simulink model "QuadcopterSimModel_LindiCopter"  (R2018b)
settings: Solver=ode23  StartTime=0.0  StopTime=1000  FixedStep=sample_time  RelTol=1e-4  EnableMultiTasking=on
undefined symbols (not defined in the file): alt_ground, atmosphere, envir, g, G10, G20, joystick, lindi, pos_ref, waypoints, wind
libraries: filters_lib x8, indi_lib x3, unit_conversions_lib x3, simulink x2, flightgear_visualization_lib x2, axes_transformation_lib x2, cntrlPosNdi_lib x2, atmosphere_lib x1, ca_lib x1, ndi_lib x1, traj_lib x1, cntrlAttiRedIndi_lib x1
settings Model: EnablePacing=on  Creator=Yannic  LastModifiedBy=yannic
settings SolverCC: ZeroCrossControl=DisableAll
settings DataIOCC: LimitDataPoints=on  ReturnWorkspaceOutputs=on
settings OptimizationCC: EfficientMapNaN2IntZero=off  LifeSpan=inf
settings DebuggingCC: ReadBeforeWriteMsg=DisableAll  WriteAfterWriteMsg=DisableAll  WriteAfterReadMsg=DisableAll  MultiTaskDSMMsg=none  AllowSymbolicDim=off  LibraryContextMissingDiagnostic=none  SFUnexpectedBacktrackingDiag=warning  SFNoUnconditionalDefaultTransitionDiag=warning  SFExecutionAtInitializationDiag=none
settings HardwareCC: TargetBitPerLong=64  TargetBitPerPointer=64  TargetBitPerSizeT=64  TargetBitPerPtrDiffT=64  TargetLongLongMode=on  TargetIntDivRoundTo=Zero  TargetEndianess=LittleEndian  TargetWordSize=64  TargetHWDeviceType=MATLAB Host  ProdEqTarget=off
settings ModelReferenceCC: UpdateModelReferenceTargets=IfOutOfDate  PropagateSignalLabelsOutOfModel=off
settings SFSimCC: SFSimEcho=off  SimUseLocalCustomCode=off
settings CodeAppCC: MaxIdLength=128
settings GRTTargetCC: TargetLangStandard=C89/C90 (ANSI)  CombineOutputUpdateFcns=off  GRTInterface=on
settings ConfigComp: CovMetricSettings=dw  CovHtmlReporting=on  CovSaveCumulativeToWorkspaceVar=on  CovSaveSingleToWorkspaceVar=on  CovExternalEMLEnable=off

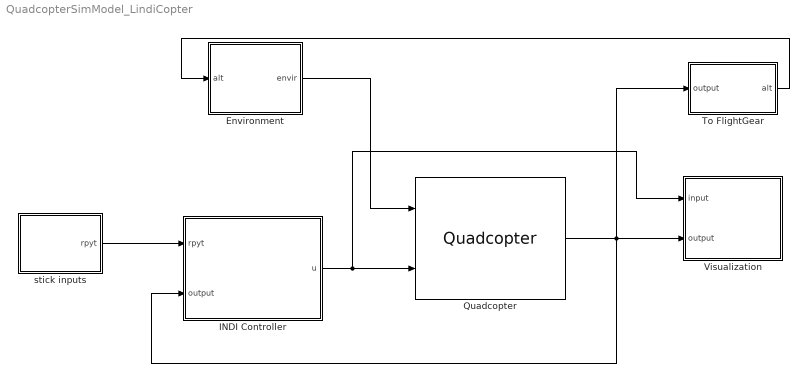
== system QuadcopterSimModel_LindiCopter ==
  Environment : Subsystem
  INDI Controller : Subsystem
  Quadcopter : quadcopter_lib/Quadcopter  copter_=copter  IC_=IC  grnd_=grnd
      settings: SourceProductName=LADAC
  To FlightGear : Subsystem
  Visualization : Subsystem
  stick inputs : Subsystem
  wires:
  Environment/1(envir) -> Quadcopter/1
  Quadcopter/1 -> To FlightGear/1(output), Visualization/2(output), INDI Controller/2(output)
  To FlightGear/1(alt) -> Environment/1(alt)
  INDI Controller/1(u) -> Quadcopter/2, Visualization/1(input)
  stick inputs/1(rpyt) -> INDI Controller/1(rpyt)

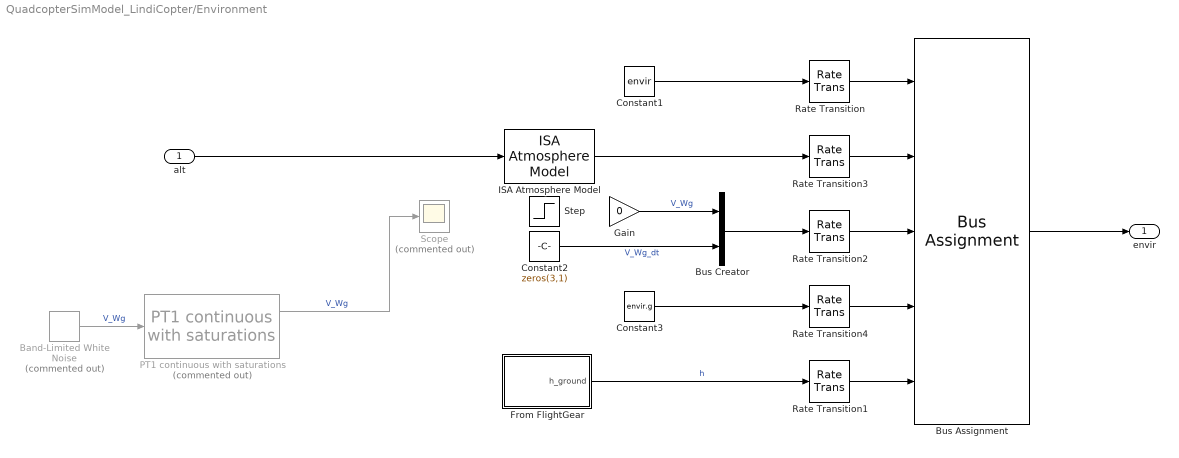
== system QuadcopterSimModel_LindiCopter/Environment ==
  alt : Inport
  Band-Limited White Noise : simulink/Sources/Band-Limited White Noise  Commented=on  Cov=10  Ts=0.0025  seed=[23341,12345,23456]
  Bus Assignment : BusAssignment  AssignedSignals=atmosphere,wind,g,alt_ground
  Bus Creator : BusCreator  Inputs=2
  Constant1 : Constant  Value=envir  OutDataTypeStr=Bus: envirBus
  Constant2 : Constant  Value=zeros(3,1)
  Constant3 : Constant  Value=envir.g
  From FlightGear : Subsystem
  Gain : Gain  Gain=0
  ISA Atmosphere Model : atmosphere_lib/ISA Atmosphere Model
      settings: SourceProductName=LADAC
  PT1 continuous with saturations : filters_lib/PT1 continuous with saturations  Commented=on  T=0.5  x_max=inf  x_min=-inf  x_dt_max=inf  x_dt_min=-inf  x_init=0
      settings: SourceProductName=LADAC
  Rate Transition{,1..4} (5 alike) : RateTransition
  Scope : Scope  Commented=on
  Step : Step  Time=5  After=[0;10;0]  SampleTime=0
  envir : Outport
  wires:
  From FlightGear/1(h_ground) -> Rate Transition1/1  "h"
  Rate Transition2/1 -> Bus Assignment/3
  Rate Transition3/1 -> Bus Assignment/2
  Bus Assignment/1 -> envir/1
  Rate Transition/1 -> Bus Assignment/1
  ISA Atmosphere Model/1 -> Rate Transition3/1
  PT1 continuous with saturations/1 -> Scope/1  "V_Wg"
  Rate Transition1/1 -> Bus Assignment/5
  Constant1/1 -> Rate Transition/1
  alt/1 -> ISA Atmosphere Model/1
  Bus Creator/1 -> Rate Transition2/1
  Constant2/1 -> Bus Creator/2  "V_Wg_dt"
  Rate Transition4/1 -> Bus Assignment/4
  Constant3/1 -> Rate Transition4/1
  Gain/1 -> Bus Creator/1  "V_Wg"
  Band-Limited White Noise/1 -> PT1 continuous with saturations/1  "V_Wg"

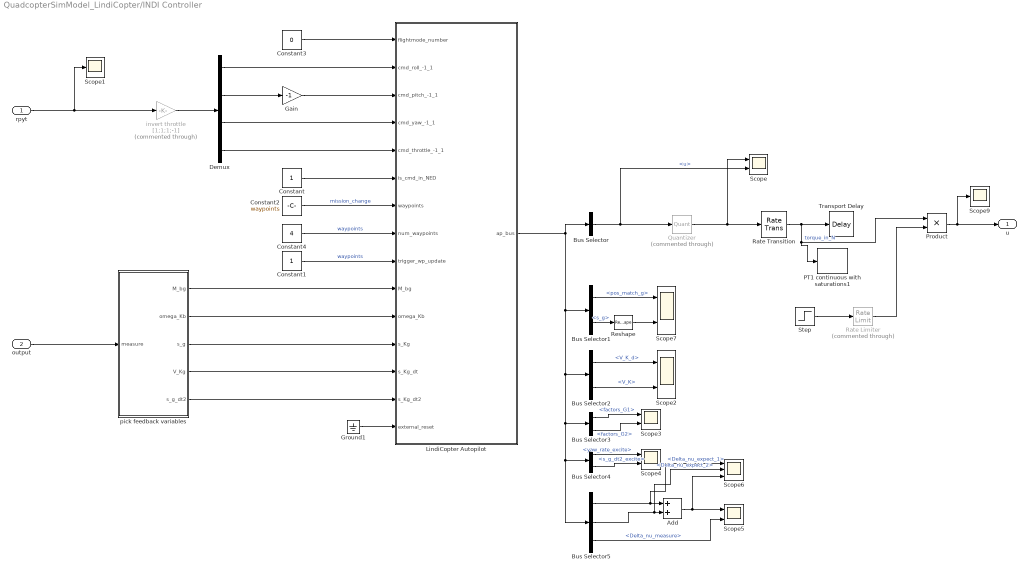
== system QuadcopterSimModel_LindiCopter/INDI Controller ==
  rpyt : Inport  OutDataTypeStr=double
  output : Inport  Port=2
  Add : Sum
  Bus Selector : BusSelector  OutputSignals=inner_loop_indi.u
  Bus Selector1 : BusSelector  OutputSignals=guidance.matching.pos_match_g,pos_cntrl.measure.s_g
  Bus Selector2 : BusSelector  OutputSignals=guidance.velocity.V_K_d,guidance.velocity.V_K
  Bus Selector3 : BusSelector  OutputSignals=autotune.factors_G1,autotune.factors_G2
  Bus Selector4 : BusSelector  OutputSignals=autotune.excite.yaw_rate_excite,autotune.excite.s_g_dt2_excite
  Bus Selector5 : BusSelector  OutputSignals=autotune.indi_inv_check.Delta_nu_expect_1,autotune.indi_inv_check.Delta_nu_expect_2,autotune.indi_inv_check.Delta_nu_measure
  Constant : Constant
  Constant1 : Constant
  Constant2 : Constant  Value=waypoints
  Constant3 : Constant  Value=0
  Constant4 : Constant  Value=4
  Demux : Demux
  Gain : Gain  Gain=-1
  Ground1 : Ground
  LindiCopter Autopilot : Subsystem  AncestorBlock=lindiCopter_lib/LindiCopter Autopilot  mask{ap=lindi}
      mask prompts: ap "LinidCopter parameters struct, see lindiCopter_params_default"
      mask init:
      | lindiCopterStateLogicBus();
      mask Help: web('hhttps://github.com/iff-gsc/LADAC/tree/main/control/autopilots/LindiCopter/README.md','-browser')
      mask DialogControl DescGroupVar Prompt: LindiCopter Autopilot
      mask DialogControl Control4 Prompt: The documentation of this block can be found here:
      mask DialogControl Control5 Prompt: README
      mask DialogControl Control5 Callback: web('https://github.com/iff-gsc/LADAC/blob/main/control/autopilots/LindiCopter/README.md','-browser')
  PT1 continuous with saturations1 : filters_lib/PT1 continuous with saturations  T=0.03  x_max=inf  x_min=-inf  x_dt_max=inf  x_dt_min=-inf  x_init=0
      settings: SourceProductName=LADAC
  Product : Product
  Quantizer : Quantizer  Commented=through  QuantizationInterval=0.001
  Rate Limiter : RateLimiter  Commented=through  RisingSlewLimit=0.3  FallingSlewLimit=-0.3  SampleTimeMode=inherited
  Rate Transition : RateTransition
  Reshape : Reshape
  Scope{,2..5,7} (6 alike) : Scope  NumInputPorts=2
  Scope1 : Scope
  Scope6 : Scope  NumInputPorts=3
  Scope9 : Scope
  Step : Step  Time=0  Before=[1;1;1;1]  After=[1;0;1;1]  SampleTime=0
  Transport Delay : TransportDelay  DelayTime=0.0025*2
  invert throttle : Gain  Commented=through  Gain=[1;1;1;-1]
  pick feedback variables : Subsystem
  u : Outport  OutDataTypeStr=double  PortDimensions=4
  wires:
  output/1 -> pick feedback variables/1(measure)
  rpyt/1 -> invert throttle/1, Scope1/1
  Bus Selector/1 -> Quantizer/1, Scope/2  "<u>"
  invert throttle/1 -> Demux/1
  LindiCopter Autopilot/1(ap_bus) -> Bus Selector/1, Bus Selector5/1, Bus Selector4/1, Bus Selector3/1, Bus Selector2/1, Bus Selector1/1
  Demux/4 -> LindiCopter Autopilot/5(cmd_throttle_-1_1)
  Demux/3 -> LindiCopter Autopilot/4(cmd_yaw_-1_1)
  Constant/1 -> LindiCopter Autopilot/6(is_cmd_in_NED)
  Ground1/1 -> LindiCopter Autopilot/15(external_reset)
  Demux/2 -> Gain/1
  Demux/1 -> LindiCopter Autopilot/2(cmd_roll_-1_1)
  Gain/1 -> LindiCopter Autopilot/3(cmd_pitch_-1_1)
  pick feedback variables/1(M_bg) -> LindiCopter Autopilot/10(M_bg)
  pick feedback variables/2(omega_Kb) -> LindiCopter Autopilot/11(omega_Kb)
  pick feedback variables/3(s_g) -> LindiCopter Autopilot/12(s_Kg)
  pick feedback variables/4(V_Kg) -> LindiCopter Autopilot/13(s_Kg_dt)
  Constant1/1 -> LindiCopter Autopilot/9(trigger_wp_update)  "waypoints"
  Constant2/1 -> LindiCopter Autopilot/7(waypoints)  "mission_change"
  Bus Selector1/2 -> Reshape/1  "<s_g>"
  Bus Selector1/1 -> Scope7/1  "<pos_match_g>"
  Bus Selector2/2 -> Scope2/2  "<V_K>"
  Bus Selector2/1 -> Scope2/1  "<V_K_d>"
  Constant3/1 -> LindiCopter Autopilot/1(flightmode_number)
  Quantizer/1 -> Rate Transition/1, Scope/1
  pick feedback variables/5(s_g_dt2) -> LindiCopter Autopilot/14(s_Kg_dt2)
  Reshape/1 -> Scope7/2
  Bus Selector3/1 -> Scope3/1  "<factors_G1>"
  Bus Selector3/2 -> Scope3/2  "<factors_G2>"
  Bus Selector4/1 -> Scope4/1  "<yaw_rate_excite>"
  Bus Selector4/2 -> Scope4/2  "<s_g_dt2_excite>"
  Bus Selector5/1 -> Scope6/1, Add/1  "<Delta_nu_expect_1>"
  Bus Selector5/2 -> Scope6/2, Add/2  "<Delta_nu_expect_2>"
  Add/1 -> Scope6/3, Scope5/1
  Bus Selector5/3 -> Scope5/2  "<Delta_nu_measure>"
  Step/1 -> Rate Limiter/1
  Constant4/1 -> LindiCopter Autopilot/8(num_waypoints)  "waypoints"
  Product/1 -> Scope9/1, u/1
  Rate Transition/1 -> Product/1, PT1 continuous with saturations1/1, Transport Delay/1  "torque_in_N"
  Rate Limiter/1 -> Product/2

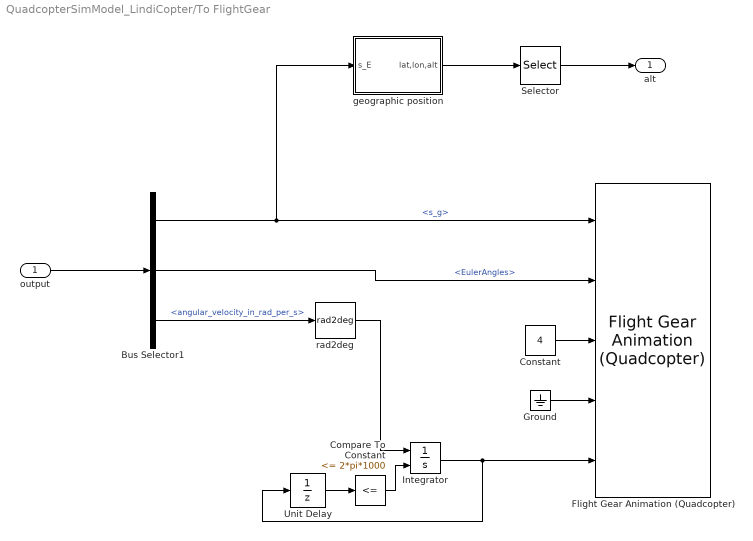
== system QuadcopterSimModel_LindiCopter/To FlightGear ==
  output : Inport
  Bus Selector1 : BusSelector  OutputSignals=rigidBodyBus.s_g,rigidBodyBus.EulerAngles,motorBus.angular_velocity_in_rad_per_s
  Compare To Constant : simulink/Logic and Bit Operations/Compare To Constant  relop=<=  const=2*pi*1000  OutDataTypeStr=boolean
  Constant : Constant  Value=4
  Flight Gear Animation (Quadcopter) : flightgear_visualization_lib/Flight Gear Animation (Quadcopter)  inital_lat=pos_ref.lat  inital_long=pos_ref.lon  inital_height=pos_ref.alt  remoteURL=fg.remoteURL  remotePort=fg.remotePort
      settings: SourceProductName=LADAC
  Ground : Ground
  Integrator : Integrator  ExternalReset=rising
  Selector : Selector  InputPortWidth=3  IndexOptions=Index vector (dialog)  Indices=3  OutputSizes=1
  Unit Delay : UnitDelay  SampleTime=-1
  geographic position : Subsystem
  rad2deg : unit_conversions_lib/rad2deg
      settings: SourceProductName=LADAC
  alt : Outport
  wires:
  Bus Selector1/1 -> geographic position/1(s_E), Flight Gear Animation (Quadcopter)/1  "<s_g>"
  output/1 -> Bus Selector1/1
  geographic position/1(lat,lon,alt) -> Selector/1
  Bus Selector1/2 -> Flight Gear Animation (Quadcopter)/2  "<EulerAngles>"
  Bus Selector1/3 -> rad2deg/1  "<angular_velocity_in_rad_per_s>"
  Selector/1 -> alt/1
  Constant/1 -> Flight Gear Animation (Quadcopter)/3
  Ground/1 -> Flight Gear Animation (Quadcopter)/4
  Integrator/1 -> Unit Delay/1, Flight Gear Animation (Quadcopter)/5
  Unit Delay/1 -> Compare To Constant/1
  Compare To Constant/1 -> Integrator/2
  rad2deg/1 -> Integrator/1

== system QuadcopterSimModel_LindiCopter/Visualization ==
  input : Inport
  output : Inport  Port=2
  Aerodynamics : Subsystem
  Bus Selector : BusSelector  OutputSignals=rigidBodyBus,aeroBus,propulsionBus,motorBus
  Motor : Subsystem
  Propulsion : Subsystem
  Scope : Scope
  rigid_body : Subsystem
  wires:
  output/1 -> Bus Selector/1
  Bus Selector/1 -> rigid_body/1(rigidBodyBus)  "<rigidBodyBus>"
  Bus Selector/2 -> Aerodynamics/1(aeroBus)  "<aeroBus>"
  Bus Selector/3 -> Propulsion/1(propulsionBus)  "<propulsionBus>"
  Bus Selector/4 -> Motor/1(motorBus)  "<motorBus>"
  input/1 -> Scope/1

== system QuadcopterSimModel_LindiCopter/stick inputs ==
  Calibrated Joystick : joystick_lib/Calibrated Joystick  jystck=joystick  joyid=1
      settings: SourceProductName=LADAC
  Constant : Constant  Value=zeros(8,1)
  Constant1 : Constant  Value=joystick.enable
  Scope : Scope
  Selector2 : Selector  InputPortWidth=8  IndexOptions=Index vector (dialog)  Indices=[1,2,3,4]  OutputSizes=1
  Switch1 : Switch  Criteria=u2 > Threshold
  rpyt : Outport
  wires:
  Constant/1 -> Switch1/3
  Switch1/1 -> Selector2/1, Scope/1
  Constant1/1 -> Calibrated Joystick/Enable, Switch1/2
  Calibrated Joystick/1 -> Switch1/1
  Selector2/1 -> rpyt/1

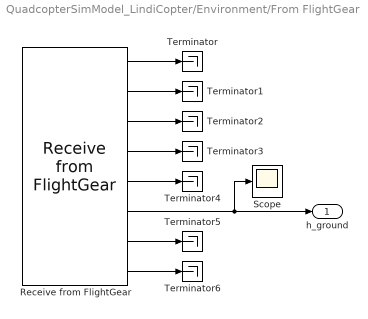
== system QuadcopterSimModel_LindiCopter/Environment/From FlightGear ==
  Receive from FlightGear : flightgear_visualization_lib/Receive from FlightGear  ip_address='127.0.0.1'  ip_port=5503  sample_time=1/30  blocking_time=0  is_aerocntrl=off  is_engine=off  is_fuel=off  is_land=off  is_avionics=off  is_envir=on
      settings: SourceProductName=LADAC
  Scope : Scope
  Terminator{,1..6} (7 alike) : Terminator
  h_ground : Outport
  wires:
  Receive from FlightGear/4 -> Terminator3/1
  Receive from FlightGear/5 -> Terminator4/1
  Receive from FlightGear/2 -> Terminator1/1
  Receive from FlightGear/7 -> Terminator5/1
  Receive from FlightGear/1 -> Terminator/1
  Receive from FlightGear/3 -> Terminator2/1
  Receive from FlightGear/8 -> Terminator6/1
  Receive from FlightGear/6 -> Scope/1, h_ground/1

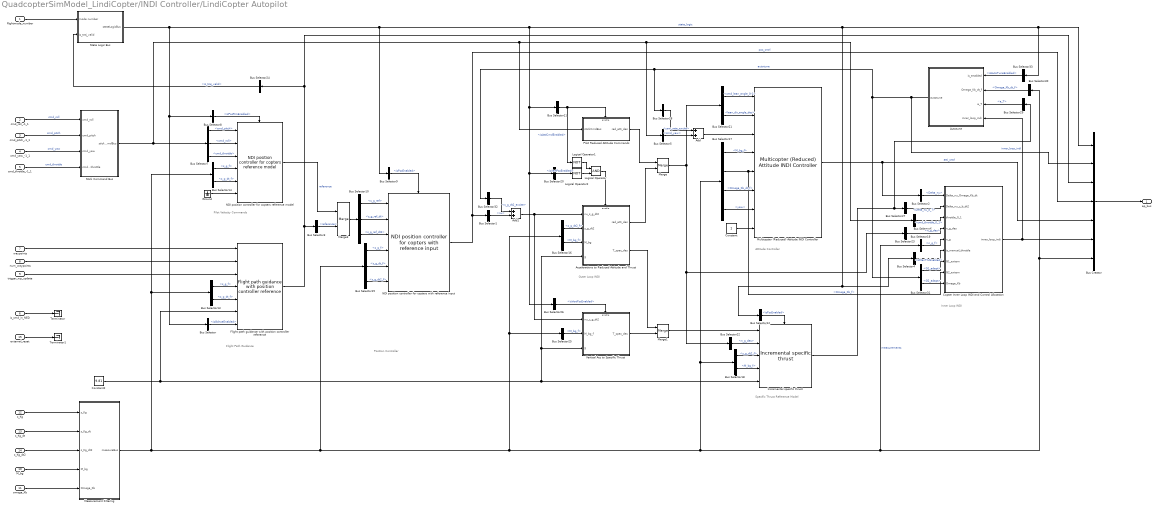
== system QuadcopterSimModel_LindiCopter/INDI Controller/LindiCopter Autopilot ==
  note: Inner Loop INDI
  note: Attitude Controller
  note: Specific Thrust
      | Reference Model
  note: Outer Loop INDI
  note: Pilot Velocity Commands
  note: Flight Path Guidance
  note: Position Controller
  flightmode_number : Inport  SampleTime=ap.ts
  cmd_roll_-1_1 : Inport  Port=2  SampleTime=ap.ts
  cmd_pitch_-1_1 : Inport  Port=3  SampleTime=ap.ts
  cmd_yaw_-1_1 : Inport  Port=4  SampleTime=ap.ts
  cmd_throttle_-1_1 : Inport  Port=5  SampleTime=ap.ts
  is_cmd_in_NED : Inport  Port=6  SampleTime=ap.ts
  waypoints : Inport  Port=7  SampleTime=ap.ts
  num_waypoints : Inport  Port=8  SampleTime=ap.ts
  trigger_wp_update : Inport  Port=9  SampleTime=ap.ts
  M_bg : Inport  Port=10  SampleTime=ap.ts
  omega_Kb : Inport  Port=11  SampleTime=ap.ts
  s_Kg : Inport  Port=12  SampleTime=ap.ts
  s_Kg_dt : Inport  Port=13  SampleTime=ap.ts
  s_Kg_dt2 : Inport  Port=14  SampleTime=ap.ts
  external_reset : Inport  Port=15  SampleTime=ap.ts
  Accelerations to Reduced Attitude and Thrust : Subsystem
  Add : Sum
  Add1 : Sum
  Autotune : Subsystem
  Bus Creator : BusCreator  Inputs=7
  Bus Selector : BusSelector  OutputSignals=isGdnceEnabled
  Bus Selector1 : BusSelector  OutputSignals=pseudo_control.nu
  Bus Selector10 : BusSelector  OutputSignals=s_g_ref,s_g_ref_dt,s_g_ref_dt2
  Bus Selector11 : BusSelector  OutputSignals=isAttiCmdEnabled
  Bus Selector12 : BusSelector  OutputSignals=isPscEnabled
  Bus Selector13 : BusSelector  OutputSignals=s_g_f,s_g_dt_f
  Bus Selector14 : BusSelector  OutputSignals=s_g_f,s_g_dt_f
  Bus Selector15 : BusSelector  OutputSignals=s_g_f,s_g_dt_f,s_g_dt2_f
  Bus Selector16 : BusSelector  OutputSignals=s_g_dt2_f,M_bg_f
  Bus Selector17 : BusSelector  OutputSignals=M_bg_f,Omega_Kb_f,Omega_Kb_dt_f,yaw
  Bus Selector18 : BusSelector  OutputSignals=s_g_dt2_f,M_bg_f
  Bus Selector19 : BusSelector  OutputSignals=n_g_f
  Bus Selector2 : BusSelector  OutputSignals=pseudo_control.Delta_ny
  Bus Selector20 : BusSelector  OutputSignals=isVertPscEnabled
  Bus Selector21 : BusSelector  OutputSignals=cmd_lean_angle_0-1,lean_dir_angle_des
  Bus Selector22 : BusSelector  OutputSignals=n_g_des
  Bus Selector23 : BusSelector  OutputSignals=n_g_des
  Bus Selector24 : BusSelector  OutputSignals=is_traj_valid
  Bus Selector25 : BusSelector  OutputSignals=M_bg_f
  Bus Selector26 : BusSelector  OutputSignals=isVertPscEnabled
  Bus Selector27 : BusSelector  OutputSignals=Delta_nu_a_T
  Bus Selector28 : BusSelector  OutputSignals=excite.yaw_rate_excite
  Bus Selector29 : BusSelector  OutputSignals=a_T
  Bus Selector3 : BusSelector  OutputSignals=reference
  Bus Selector30 : BusSelector  OutputSignals=Omega_Kb_dt_f
  Bus Selector31 : BusSelector  OutputSignals=G1_adapt,G2_adapt
  Bus Selector32 : BusSelector  OutputSignals=excite.s_g_dt2_excite
  Bus Selector33 : BusSelector  OutputSignals=isAutoTuneEnabled
  Bus Selector4 : BusSelector  OutputSignals=isManThrEnabled
  Bus Selector5 : BusSelector  OutputSignals=cmd_yaw
  Bus Selector6 : BusSelector  OutputSignals=cmd_throttle_0_1
  Bus Selector7 : BusSelector  OutputSignals=cmd_pitch,cmd_roll,cmd_throttle
  Bus Selector8 : BusSelector  OutputSignals=isPosRmEnabled
  Bus Selector9 : BusSelector  OutputSignals=isPscEnabled
  Constant : Constant
  Constant2 : Constant  Value=9.81
  Copter Inner Loop INDI and Control Allocation : Subsystem  AncestorBlock=indi_lib/Copter Inner Loop INDI and Control Allocation  mask{cep=ap.cep, ceb=ap.ceb, ca=ap.ca, mtc=ap.mtc, sflt=ap.sflt, ts=ap.ts, is_ce_extern=on}
      mask prompts: cep "Parameters for motor-propeller control effectiveness, see indiCeProp_params_default"; ceb "Parameters for body control effectiveness, see indiCeBody_params_default"; ca "Control allocation parameters, see controlAllocationWlsLoadParams"; mtc "Motor time constant, s"; sflt "Sensor filter parameters, see indiSensFiltLoadParams"; ts "Sample time, s"; is_ce_extern "Enable external control effectiveness"
      mask init:
      | caIndiCopterBlockInit(is_ce_extern);
      mask DialogControl DescGroupVar Prompt: Copter Inner Loop INDI and Control Allocation
  Flight path guidance with position controller reference : traj_lib/Flight path guidance with position controller reference  traj_params=ap.traj  T_inner_loop=2./ap.atc.rm.leanfreq + ap.mtc + 2./ap.sflt.omega
      settings: SourceProductName=LADAC
  Ground : Ground
  Incremental specific thrust : indi_lib/Incremental specific thrust  leanfreq=ap.atc.rm.leanfreq  leandamp=ap.atc.rm.leandamp  is_enable_checked=on  states_when_enabling=held
      settings: SourceProductName=LADAC
  Logical Operator : Logic  AllPortsSameDT=off  OutDataTypeStr=boolean
  Logical Operator1 : Logic  Operator=NOT  AllPortsSameDT=off  OutDataTypeStr=boolean
  Logical Operator2 : Logic  Operator=NOT  AllPortsSameDT=off  OutDataTypeStr=boolean
  Measurement Filtering : Subsystem
  Merge : Merge
  Merge1 : Merge
  Merge3 : Merge
  Multicopter (Reduced) Attitude INDI Controller : cntrlAttiRedIndi_lib/Multicopter (Reduced) Attitude INDI Controller  atc=ap.atc  T=ap.mtc + 2./ap.sflt.omega
      settings: SourceProductName=LADAC
  NDI position controller for copters reference model : cntrlPosNdi_lib/NDI position controller for copters reference model  psc=ap.psc  is_enable_checked=on  states_when_enabling=reset
      settings: SourceProductName=LADAC
  NDI position controller for copters with reference input : cntrlPosNdi_lib/NDI position controller for copters with reference input  psc=ap.psc  T_inner_loop=2./ap.atc.rm.leanfreq + ap.mtc + 2./ap.sflt.omega  is_enable_checked=on  states_when_enabling=held
      settings: SourceProductName=LADAC
  Pilot Reduced Attitude Commands : Subsystem
  State Logic Bus : Subsystem
  Stick Command Bus : Subsystem
  Terminator : Terminator
  Terminator1 : Terminator
  Vertical Acc to Specific Thrust : Subsystem
  ap_bus : Outport  SampleTime=ap.ts
  wires:
  num_waypoints/1 -> Flight path guidance with position controller reference/2
  Bus Selector5/1 -> Add/2  "<cmd_yaw>"
  Bus Selector33/1 -> Autotune/1(is_enabled)  "<isAutoTuneEnabled>"
  Bus Selector32/1 -> Add1/1  "<s_g_dt2_excite>"
  Bus Selector28/1 -> Add/1  "<yaw_rate_excite>"
  Autotune/1(autotune) -> Bus Selector32/1, Bus Selector28/1, Bus Selector31/1, Bus Creator/2  "autotune"
  Bus Selector29/1 -> Autotune/3(a_T)  "<a_T>"
  Bus Selector30/1 -> Autotune/2(Omega_Kb_dt_f)  "<Omega_Kb_dt_f>"
  Bus Selector31/1 -> Copter Inner Loop INDI and Control Allocation/7(G1_extern)  "<G1_adapt>"
  Bus Selector31/2 -> Copter Inner Loop INDI and Control Allocation/8(G2_extern)  "<G2_adapt>"
  Bus Selector27/1 -> Copter Inner Loop INDI and Control Allocation/2(Delta_nu_z_b_dt2)  "<Delta_nu_a_T>"
  Logical Operator/1 -> Accelerations to Reduced Attitude and Thrust/Enable
  Logical Operator2/1 -> Logical Operator/2
  Logical Operator1/1 -> Logical Operator/1
  Bus Selector26/1 -> Vertical Acc to Specific Thrust/Enable  "<isVertPscEnabled>"
  Bus Selector25/1 -> Vertical Acc to Specific Thrust/2(M_bg_f)  "<M_bg_f>"
  Vertical Acc to Specific Thrust/1(T_spec_des) -> Merge1/2
  Accelerations to Reduced Attitude and Thrust/2(T_spec_des) -> Merge1/1
  Accelerations to Reduced Attitude and Thrust/1(red_atti_des) -> Merge/2
  Bus Selector23/1 -> Copter Inner Loop INDI and Control Allocation/4(n_g_des)  "<n_g_des>"
  Pilot Reduced Attitude Commands/1(red_atti_des) -> Merge/1
  Merge/1 -> Bus Selector23/1, Bus Selector22/1, Bus Selector21/1
  Bus Selector21/2 -> Multicopter (Reduced) Attitude INDI Controller/2  "<lean_dir_angle_des>"
  Bus Selector21/1 -> Multicopter (Reduced) Attitude INDI Controller/1  "<cmd_lean_angle_0-1>"
  cmd_throttle_-1_1/1 -> Stick Command Bus/4(cmd_throttle)  "cmd_throttle"
  cmd_yaw_-1_1/1 -> Stick Command Bus/3(cmd_yaw)  "cmd_yaw"
  cmd_pitch_-1_1/1 -> Stick Command Bus/2(cmd_pitch)  "cmd_pitch"
  cmd_roll_-1_1/1 -> Stick Command Bus/1(cmd_roll)  "cmd_roll"
  Stick Command Bus/1(stickCmdBus) -> Bus Selector7/1, Bus Selector5/1, Bus Selector6/1, Pilot Reduced Attitude Commands/1(stickCmdBus)
  Bus Selector17/4 -> Multicopter (Reduced) Attitude INDI Controller/7  "<yaw>"
  Bus Selector19/1 -> Copter Inner Loop INDI and Control Allocation/5(n_g)  "<n_g_f>"
  Bus Selector22/1 -> Incremental specific thrust/2  "<n_g_des>"
  Bus Selector18/2 -> Incremental specific thrust/4  "<M_bg_f>"
  Bus Selector18/1 -> Incremental specific thrust/3  "<s_g_dt2_f>"
  Bus Selector17/3 -> Multicopter (Reduced) Attitude INDI Controller/6  "<Omega_Kb_dt_f>"
  Bus Selector17/2 -> Copter Inner Loop INDI and Control Allocation/9(Omega_Kb), Multicopter (Reduced) Attitude INDI Controller/5  "<Omega_Kb_f>"
  Bus Selector17/1 -> Multicopter (Reduced) Attitude INDI Controller/4  "<M_bg_f>"
  Bus Selector16/2 -> Accelerations to Reduced Attitude and Thrust/3(M_bg)  "<M_bg_f>"
  Bus Selector16/1 -> Accelerations to Reduced Attitude and Thrust/2(s_g_dt2)  "<s_g_dt2_f>"
  Bus Selector15/3 -> NDI position controller for copters with reference input/6  "<s_g_dt2_f>"
  Bus Selector15/2 -> NDI position controller for copters with reference input/5  "<s_g_dt_f>"
  Bus Selector15/1 -> NDI position controller for copters with reference input/4  "<s_g_f>"
  Bus Selector14/2 -> NDI position controller for copters reference model/5  "<s_g_dt_f>"
  Bus Selector14/1 -> NDI position controller for copters reference model/4  "<s_g_f>"
  Bus Selector13/2 -> Flight path guidance with position controller reference/5  "<s_g_dt_f>"
  Bus Selector13/1 -> Flight path guidance with position controller reference/4  "<s_g_f>"
  Measurement Filtering/1(measureBus) -> Bus Selector13/1, Bus Selector14/1, Bus Selector17/1, Bus Selector18/1, Bus Creator/7, Bus Selector30/1, Bus Selector19/1, Bus Selector25/1, Bus Selector16/1, Bus Selector15/1  "measurements"
  Ground/1 -> NDI position controller for copters reference model/6
  Bus Selector12/1 -> Incremental specific thrust/Enable  "<isPscEnabled>"
  Bus Selector11/1 -> Pilot Reduced Attitude Commands/Enable, Logical Operator1/1  "<isAttiCmdEnabled>"
  Bus Selector9/1 -> NDI position controller for copters with reference input/Enable  "<isPscEnabled>"
  Bus Selector8/1 -> NDI position controller for copters reference model/Enable  "<isPosRmEnabled>"
  Bus Selector/1 -> Flight path guidance with position controller reference/7  "<isGdnceEnabled>"
  trigger_wp_update/1 -> Flight path guidance with position controller reference/3
  waypoints/1 -> Flight path guidance with position controller reference/1
  Flight path guidance with position controller reference/1 -> Bus Selector3/1, Bus Selector24/1, Bus Creator/3
  Bus Selector7/2 -> NDI position controller for copters reference model/2  "<cmd_roll>"
  Bus Selector7/1 -> NDI position controller for copters reference model/1  "<cmd_pitch>"
  Bus Selector7/3 -> NDI position controller for copters reference model/3  "<cmd_throttle>"
  Bus Selector6/1 -> Copter Inner Loop INDI and Control Allocation/3(throttle_0_1)  "<cmd_throttle_0_1>"
  Add/1 -> Multicopter (Reduced) Attitude INDI Controller/3
  Bus Selector4/1 -> Copter Inner Loop INDI and Control Allocation/6(is_manual_throttle)  "<isManThrEnabled>"
  State Logic Bus/1(stateLogicBus) -> Bus Creator/1, Bus Selector33/1, Bus Selector4/1, Bus Selector12/1, Bus Selector11/1, Bus Selector20/1, Bus Selector26/1, Bus Selector9/1, Bus Selector/1, Bus Selector8/1  "state_logic"
  s_Kg/1 -> Measurement Filtering/1(s_Kg)
  s_Kg_dt/1 -> Measurement Filtering/2(s_Kg_dt)
  s_Kg_dt2/1 -> Measurement Filtering/3(s_Kg_dt2)
  M_bg/1 -> Measurement Filtering/4(M_bg)
  omega_Kb/1 -> Measurement Filtering/5(Omega_Kb)
  Incremental specific thrust/1 -> Bus Selector29/1, Bus Selector27/1
  Merge1/1 -> Incremental specific thrust/1
  external_reset/1 -> Terminator1/1
  flightmode_number/1 -> State Logic Bus/1(mode number)
  NDI position controller for copters reference model/1 -> Merge3/1  "reference"
  Constant2/1 -> Accelerations to Reduced Attitude and Thrust/4(g), Vertical Acc to Specific Thrust/3(g), Incremental specific thrust/5, Flight path guidance with position controller reference/6
  Bus Selector10/1 -> NDI position controller for copters with reference input/1  "<s_g_ref>"
  Bus Selector10/2 -> NDI position controller for copters with reference input/2  "<s_g_ref_dt>"
  Bus Selector10/3 -> NDI position controller for copters with reference input/3  "<s_g_ref_dt2>"
  Constant/1 -> Multicopter (Reduced) Attitude INDI Controller/8
  NDI position controller for copters with reference input/1 -> Bus Creator/4, Bus Selector1/1  "pos_cntrl"
  Bus Selector1/1 -> Add1/2  "<nu>"
  Bus Creator/1 -> ap_bus/1
  is_cmd_in_NED/1 -> Terminator/1
  Multicopter (Reduced) Attitude INDI Controller/1 -> Bus Creator/5, Bus Selector2/1  "atti_cntrl"
  Copter Inner Loop INDI and Control Allocation/1(inner_loop_indi) -> Bus Creator/6, Autotune/4(inner_loop_indi)  "inner_loop_indi"
  Bus Selector2/1 -> Copter Inner Loop INDI and Control Allocation/1(Delta_nu_Omega_Kb_dt)  "<Delta_ny>"
  Bus Selector20/1 -> Logical Operator2/1  "<isVertPscEnabled>"
  Merge3/1 -> Bus Selector10/1
  Bus Selector3/1 -> Merge3/2  "<reference>"
  Add1/1 -> Accelerations to Reduced Attitude and Thrust/1(nu_s_g_dt2), Vertical Acc to Specific Thrust/1(nu_z_g_dt2)
  Bus Selector24/1 -> State Logic Bus/2(is_traj_valid)  "<is_traj_valid>"

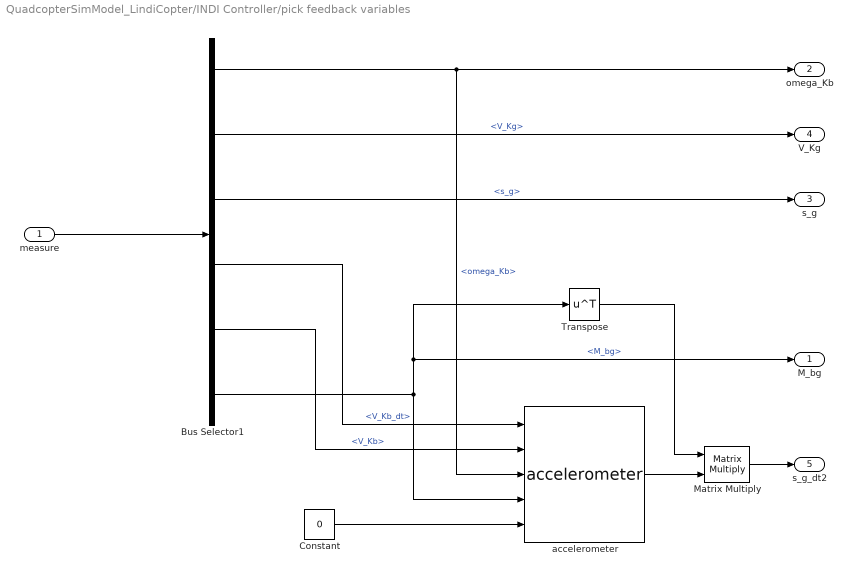
== system QuadcopterSimModel_LindiCopter/INDI Controller/pick feedback variables ==
  measure : Inport
  Bus Selector1 : BusSelector  OutputSignals=rigidBodyBus.omega_Kb,rigidBodyBus.V_Kg,rigidBodyBus.s_g,rigidBodyBus.V_Kb_dt,rigidBodyBus.V_Kb,rigidBodyBus.M_bg
  Constant : Constant  Value=0  OutDataTypeStr=Inherit: Inherit via back propagation
  Matrix Multiply : Product  Multiplication=Matrix(*)
  Transpose : Math  Operator=transpose  SaturateOnIntegerOverflow=on
  accelerometer : sensors_lib/accelerometer  SystemSampleTime=-1
      settings: SourceProductName=LADAC
  M_bg : Outport
  omega_Kb : Outport  Port=2
  s_g : Outport  Port=3
  V_Kg : Outport  Port=4
  s_g_dt2 : Outport  Port=5
  wires:
  measure/1 -> Bus Selector1/1
  Bus Selector1/2 -> V_Kg/1  "<V_Kg>"
  Constant/1 -> accelerometer/5
  accelerometer/1 -> Matrix Multiply/2
  Matrix Multiply/1 -> s_g_dt2/1
  Transpose/1 -> Matrix Multiply/1
  Bus Selector1/1 -> accelerometer/3, omega_Kb/1  "<omega_Kb>"
  Bus Selector1/3 -> s_g/1  "<s_g>"
  Bus Selector1/5 -> accelerometer/2  "<V_Kb>"
  Bus Selector1/4 -> accelerometer/1  "<V_Kb_dt>"
  Bus Selector1/6 -> M_bg/1, Transpose/1, accelerometer/4  "<M_bg>"

== system QuadcopterSimModel_LindiCopter/To FlightGear/geographic position ==
  s_E : Inport
  Constant : Constant  Value=pos_ref.lat
  Constant1 : Constant  Value=pos_ref.lon
  Constant2 : Constant  Value=pos_ref.alt
  Mux : Mux  Inputs=3
  Scope : Scope  NumInputPorts=3
  "flat earth to lat, lon, alt" : axes_transformation_lib/NED to lat, lon, alt  SystemSampleTime=-1
      settings: SourceProductName=LADAC
  lat,lon,alt : Outport
  wires:
  Constant2/1 -> "flat earth to lat, lon, alt"/3
  Constant1/1 -> "flat earth to lat, lon, alt"/2
  "flat earth to lat, lon, alt"/3 -> Scope/3, Mux/3
  Constant/1 -> "flat earth to lat, lon, alt"/1
  Mux/1 -> lat,lon,alt/1
  s_E/1 -> "flat earth to lat, lon, alt"/4
  "flat earth to lat, lon, alt"/2 -> Mux/2, Scope/2
  "flat earth to lat, lon, alt"/1 -> Mux/1, Scope/1

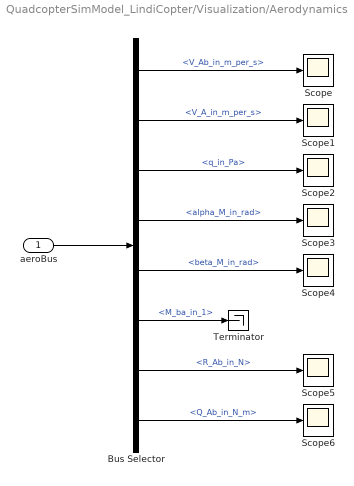
== system QuadcopterSimModel_LindiCopter/Visualization/Aerodynamics ==
  aeroBus : Inport
  Bus Selector : BusSelector  OutputSignals=V_Ab_in_m_per_s,V_A_in_m_per_s,q_in_Pa,angles.alpha_M_in_rad,angles.beta_M_in_rad,M_ba_in_1,R_Ab_in_N,Q_Ab_in_N_m
  Scope{,1..6} (7 alike) : Scope
  Terminator : Terminator
  wires:
  aeroBus/1 -> Bus Selector/1
  Bus Selector/1 -> Scope/1  "<V_Ab_in_m_per_s>"
  Bus Selector/2 -> Scope1/1  "<V_A_in_m_per_s>"
  Bus Selector/3 -> Scope2/1  "<q_in_Pa>"
  Bus Selector/4 -> Scope3/1  "<alpha_M_in_rad>"
  Bus Selector/5 -> Scope4/1  "<beta_M_in_rad>"
  Bus Selector/6 -> Terminator/1  "<M_ba_in_1>"
  Bus Selector/7 -> Scope5/1  "<R_Ab_in_N>"
  Bus Selector/8 -> Scope6/1  "<Q_Ab_in_N_m>"

== system QuadcopterSimModel_LindiCopter/Visualization/Motor ==
  motorBus : Inport
  Bus Selector : BusSelector  OutputSignals=angular_acceleration_in_rad_per_square_s,angular_velocity_in_rad_per_s
  Scope : Scope
  Scope1 : Scope
  wires:
  Bus Selector/1 -> Scope/1  "<angular_acceleration_in_rad_per_square_s>"
  motorBus/1 -> Bus Selector/1
  Bus Selector/2 -> Scope1/1  "<angular_velocity_in_rad_per_s>"

== system QuadcopterSimModel_LindiCopter/Visualization/Propulsion ==
  propulsionBus : Inport
  Bus Selector : BusSelector  OutputSignals=propeller_1.thrust_in_N,propeller_2.thrust_in_N,propeller_3.thrust_in_N,propeller_4.thrust_in_N,propeller_1.torque_in_N,propeller_2.torque_in_N,propeller_3.torque_in_N,propeller_4.torque_in_N,propeller_1.R_Fb_in_N,propeller_2.R_Fb_in_N,propeller_3.R_Fb_in_N,propeller_4.R_Fb_in_N,propeller_1.Q_Fb_in_Nm,propeller_2.Q_Fb_in_Nm,propeller_3.Q_Fb_in_Nm,propeller_4.Q_Fb_in_Nm,propeller_1.V_A_prop_in_m_per_s,propeller_2.V_A_prop_in_m_per_s,propeller_3.V_A_prop_in_m_per_s,propeller_4.V_A_prop_in_m_per_s,R_Fb_in_N,Q_Fb_in_N
  Q_Fb : Scope  NumInputPorts=4
  R_Fb : Scope  NumInputPorts=4
  Scope5 : Scope
  Scope6 : Scope
  V_A_prop : Scope  NumInputPorts=4
  thrust : Scope  NumInputPorts=4
  torque : Scope  NumInputPorts=4
  wires:
  propulsionBus/1 -> Bus Selector/1
  Bus Selector/1 -> thrust/1  "<thrust_in_N>"
  Bus Selector/2 -> thrust/2  "<thrust_in_N>"
  Bus Selector/3 -> thrust/3  "<thrust_in_N>"
  Bus Selector/4 -> thrust/4  "<thrust_in_N>"
  Bus Selector/5 -> torque/1  "<torque_in_N>"
  Bus Selector/6 -> torque/2  "<torque_in_N>"
  Bus Selector/7 -> torque/3  "<torque_in_N>"
  Bus Selector/8 -> torque/4  "<torque_in_N>"
  Bus Selector/9 -> R_Fb/1  "<R_Fb_in_N>"
  Bus Selector/10 -> R_Fb/2  "<R_Fb_in_N>"
  Bus Selector/11 -> R_Fb/3  "<R_Fb_in_N>"
  Bus Selector/12 -> R_Fb/4  "<R_Fb_in_N>"
  Bus Selector/13 -> Q_Fb/1  "<Q_Fb_in_Nm>"
  Bus Selector/14 -> Q_Fb/2  "<Q_Fb_in_Nm>"
  Bus Selector/15 -> Q_Fb/3  "<Q_Fb_in_Nm>"
  Bus Selector/16 -> Q_Fb/4  "<Q_Fb_in_Nm>"
  Bus Selector/17 -> V_A_prop/1  "<V_A_prop_in_m_per_s>"
  Bus Selector/18 -> V_A_prop/2  "<V_A_prop_in_m_per_s>"
  Bus Selector/19 -> V_A_prop/3  "<V_A_prop_in_m_per_s>"
  Bus Selector/20 -> V_A_prop/4  "<V_A_prop_in_m_per_s>"
  Bus Selector/21 -> Scope5/1  "<R_Fb_in_N>"
  Bus Selector/22 -> Scope6/1  "<Q_Fb_in_N>"

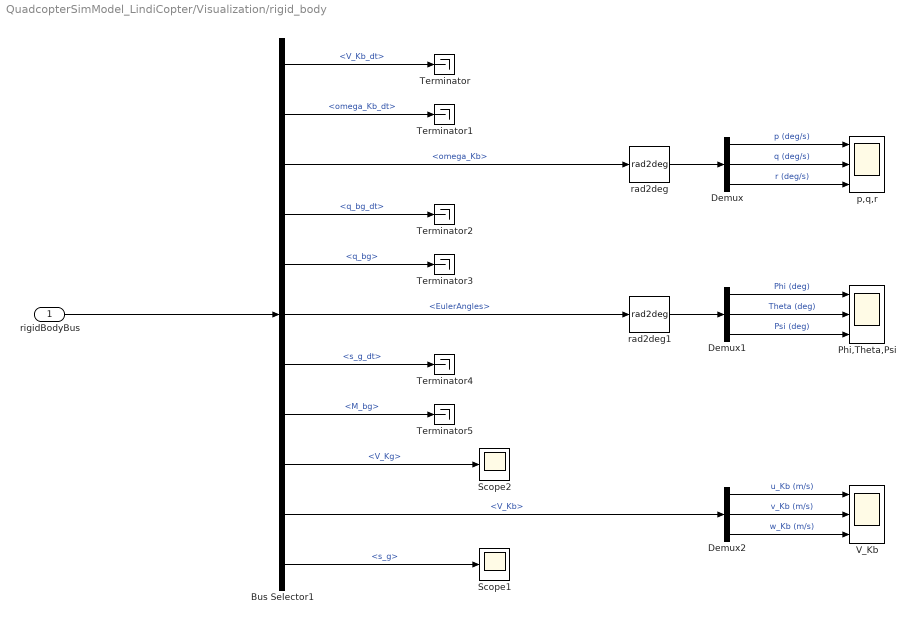
== system QuadcopterSimModel_LindiCopter/Visualization/rigid_body ==
  rigidBodyBus : Inport
  Bus Selector1 : BusSelector  OutputSignals=V_Kb_dt,omega_Kb_dt,omega_Kb,q_bg_dt,q_bg,EulerAngles,s_g_dt,M_bg,V_Kg,V_Kb,s_g
  Demux : Demux  Outputs=3
  Demux1 : Demux  Outputs=3
  Demux2 : Demux  Outputs=3
  Phi,Theta,Psi : Scope  NumInputPorts=3
  Scope1 : Scope
  Scope2 : Scope
  Terminator{,1..5} (6 alike) : Terminator
  V_Kb : Scope  NumInputPorts=3
  p,q,r : Scope  NumInputPorts=3
  rad2deg : unit_conversions_lib/rad2deg
      settings: SourceProductName=LADAC
  rad2deg1 : unit_conversions_lib/rad2deg
      settings: SourceProductName=LADAC
  wires:
  Demux/1 -> p,q,r/1  "p (deg/s)"
  Demux1/2 -> Phi,Theta,Psi/2  "Theta (deg)"
  rad2deg/1 -> Demux/1
  Demux1/1 -> Phi,Theta,Psi/1  "Phi (deg)"
  Demux1/3 -> Phi,Theta,Psi/3  "Psi (deg)"
  Demux2/3 -> V_Kb/3  "w_Kb (m/s)"
  Bus Selector1/7 -> Terminator4/1  "<s_g_dt>"
  Bus Selector1/6 -> rad2deg1/1  "<EulerAngles>"
  Bus Selector1/3 -> rad2deg/1  "<omega_Kb>"
  Demux/3 -> p,q,r/3  "r (deg/s)"
  Bus Selector1/1 -> Terminator/1  "<V_Kb_dt>"
  Demux2/2 -> V_Kb/2  "v_Kb (m/s)"
  Demux/2 -> p,q,r/2  "q (deg/s)"
  rad2deg1/1 -> Demux1/1
  Bus Selector1/5 -> Terminator3/1  "<q_bg>"
  Demux2/1 -> V_Kb/1  "u_Kb (m/s)"
  Bus Selector1/10 -> Demux2/1  "<V_Kb>"
  rigidBodyBus/1 -> Bus Selector1/1
  Bus Selector1/8 -> Terminator5/1  "<M_bg>"
  Bus Selector1/4 -> Terminator2/1  "<q_bg_dt>"
  Bus Selector1/2 -> Terminator1/1  "<omega_Kb_dt>"
  Bus Selector1/9 -> Scope2/1  "<V_Kg>"
  Bus Selector1/11 -> Scope1/1  "<s_g>"

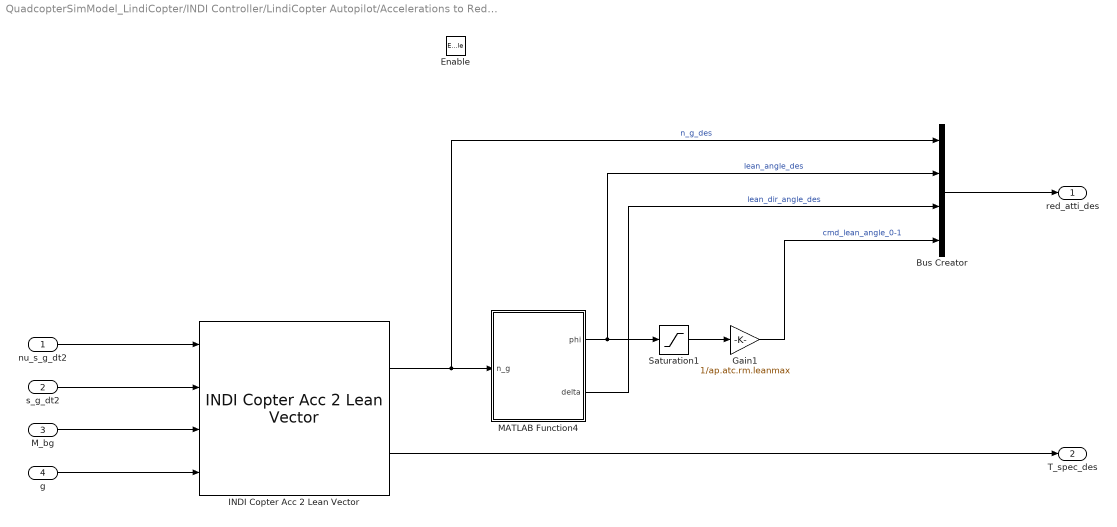
== system QuadcopterSimModel_LindiCopter/INDI Controller/LindiCopter Autopilot/Accelerations to Reduced Attitude and Thrust ==
  nu_s_g_dt2 : Inport
  s_g_dt2 : Inport  Port=2
  M_bg : Inport  Port=3
  g : Inport  Port=4
  Enable : EnablePort
  Bus Creator : BusCreator  Inputs=4
  Gain1 : Gain  Gain=1/ap.atc.rm.leanmax
  INDI Copter Acc 2 Lean Vector : indi_lib/INDI Copter Acc 2 Lean Vector  SystemSampleTime=-1
      settings: SourceProductName=LADAC
  MATLAB Function4 : MATLAB Function  TreatAsAtomicUnit=on
  Saturation1 : Saturate  UpperLimit=ap.atc.rm.leanmax  LowerLimit=0
  red_atti_des : Outport
  T_spec_des : Outport  Port=2
  wires:
  Bus Creator/1 -> red_atti_des/1
  INDI Copter Acc 2 Lean Vector/2 -> T_spec_des/1
  INDI Copter Acc 2 Lean Vector/1 -> MATLAB Function4/1(n_g), Bus Creator/1  "n_g_des"
  M_bg/1 -> INDI Copter Acc 2 Lean Vector/3
  s_g_dt2/1 -> INDI Copter Acc 2 Lean Vector/2
  g/1 -> INDI Copter Acc 2 Lean Vector/4
  MATLAB Function4/1(phi) -> Saturation1/1, Bus Creator/2  "lean_angle_des"
  Saturation1/1 -> Gain1/1
  nu_s_g_dt2/1 -> INDI Copter Acc 2 Lean Vector/1
  Gain1/1 -> Bus Creator/4  "cmd_lean_angle_0-1"
  MATLAB Function4/2(delta) -> Bus Creator/3  "lean_dir_angle_des"

== system QuadcopterSimModel_LindiCopter/INDI Controller/LindiCopter Autopilot/Autotune ==
  is_enabled : Inport
  Omega_Kb_dt_f : Inport  Port=2
  a_T : Inport  Port=3
  inner_loop_indi : Inport  Port=4
  Bus Selector28 : BusSelector  OutputSignals=G1,G2,u_bar_f,u_bar_f_dt
  Copter INDI Autotune : indi_lib/Copter INDI Autotune  rm_atc=ap.atc.rm  mtc=ap.mtc  sflt_omega=ap.sflt.omega  ts=ap.ts
      settings: SourceProductName=LADAC
  autotune : Outport
  wires:
  Omega_Kb_dt_f/1 -> Copter INDI Autotune/5
  a_T/1 -> Copter INDI Autotune/6
  Copter INDI Autotune/1 -> autotune/1
  Bus Selector28/3 -> Copter INDI Autotune/3  "<u_bar_f>"
  Bus Selector28/1 -> Copter INDI Autotune/1  "<G1>"
  inner_loop_indi/1 -> Bus Selector28/1
  Bus Selector28/2 -> Copter INDI Autotune/2  "<G2>"
  Bus Selector28/4 -> Copter INDI Autotune/4  "<u_bar_f_dt>"
  is_enabled/1 -> Copter INDI Autotune/7

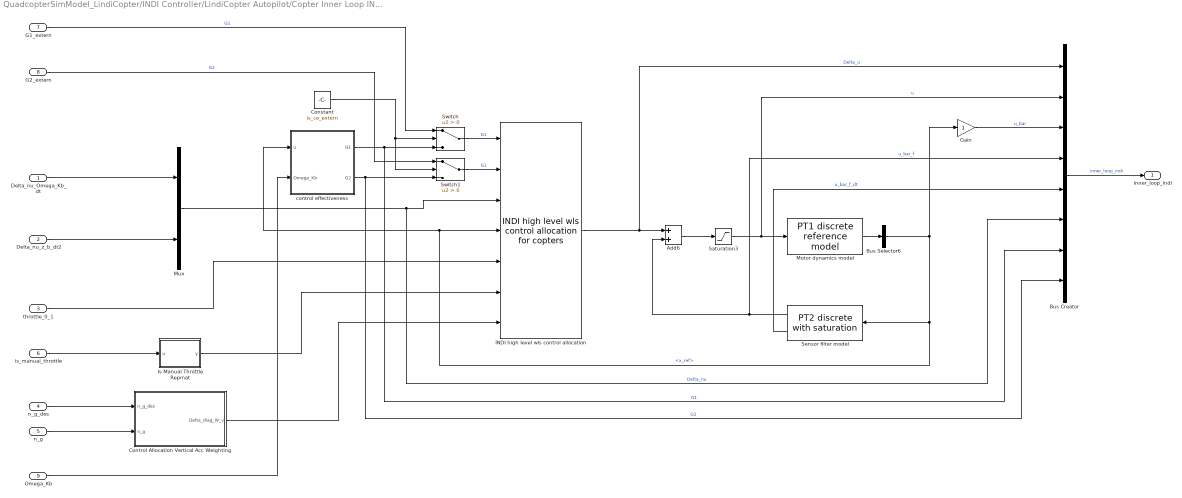
== system QuadcopterSimModel_LindiCopter/INDI Controller/LindiCopter Autopilot/Copter Inner Loop INDI and Control Allocation ==
  Delta_nu_Omega_Kb_dt : Inport
  Delta_nu_z_b_dt2 : Inport  Port=2
  throttle_0_1 : Inport  Port=3
  n_g_des : Inport  Port=4
  n_g : Inport  Port=5
  is_manual_throttle : Inport  Port=6
  G1_extern : Inport  Port=7
  G2_extern : Inport  Port=8
  Omega_Kb : Inport  Port=9
  Add6 : Sum
  Bus Creator : BusCreator  Inputs=8
  Bus Selector6 : BusSelector  OutputSignals=x_ref
  Constant : Constant  Value=is_ce_extern
  Control Allocation Vertical Acc Weighting : MATLAB Function  TreatAsAtomicUnit=on
  Gain : Gain
  INDI high level wls control allocation : ca_lib/INDI high level wls control allocation for copters  ca=ca  is_Delta_W_v_check=on  is_W_check=off  is_iter_check=off
      settings: SourceProductName=LADAC
  Is Manual Throttle Repmat : MATLAB Function  TreatAsAtomicUnit=on
  Motor dynamics model : ndi_lib/PT1 discrete reference model  T=mtc  x_max=inf  x_min=-inf  x_dt_max=inf  x_dt_min=-inf  x_init=0
      settings: SourceProductName=LADAC
  Mux : Mux  Inputs=2
  Saturation3 : Saturate  UpperLimit=ca.u_max  LowerLimit=ca.u_min
  Sensor filter model : filters_lib/PT2 discrete with saturation  param_src=internal  omega=sflt.omega  d=sflt.D  x_dt2_max=inf  x_dt2_min=-inf  x_dt_max=inf  x_dt_min=-inf  x_max=inf  x_min=-inf  y_0_src=internal  x_init=0  y_dt_0_src=internal  x_dt_init=0  is_y_dt_checked=on  is_y_dt2_checked=off
      settings: SourceProductName=LADAC
  Switch : Switch  Criteria=u2 > Threshold
  Switch1 : Switch  Criteria=u2 > Threshold
  control effectiveness : Subsystem  mask{cep=cep, ceb=ceb, ts=ts, u_min=ca.u_min}
      mask prompts: cep "propeller control effectiveness struct, see cntrlEffectPropLoadParams"; ceb "body control effectiveness struct, see cntrlEffectBodyLoadParams"; ts "controller sample time, s"
      mask init:
      | [G10,G20] = indiCePropFix( cep, ceb, ts );
  inner_loop_indi : Outport
  wires:
  Sensor filter model/2 -> Bus Creator/5  "u_bar_f_dt"
  Constant/1 -> Switch/2, Switch1/2
  G2_extern/1 -> Switch1/1  "G2"
  G1_extern/1 -> Switch/1  "G1"
  Switch1/1 -> INDI high level wls control allocation/2  "G1"
  Switch/1 -> INDI high level wls control allocation/1  "G1"
  Sensor filter model/1 -> Bus Creator/4, Add6/2  "u_bar_f"
  Mux/1 -> INDI high level wls control allocation/3, Bus Creator/6  "Delta_nu"
  Saturation3/1 -> Bus Creator/2, Motor dynamics model/1  "u"
  INDI high level wls control allocation/1 -> Bus Creator/1, Add6/1  "Delta_u"
  throttle_0_1/1 -> INDI high level wls control allocation/5
  Bus Selector6/1 -> Gain/1, Sensor filter model/1, INDI high level wls control allocation/4, control effectiveness/1(u)  "<x_ref>"
  control effectiveness/1(G1) -> Switch/3, Bus Creator/7  "G1"
  is_manual_throttle/1 -> Is Manual Throttle Repmat/1(u)
  Motor dynamics model/1 -> Bus Selector6/1
  Add6/1 -> Saturation3/1
  Delta_nu_Omega_Kb_dt/1 -> Mux/1
  control effectiveness/2(G2) -> Bus Creator/8, Switch1/3  "G2"
  Delta_nu_z_b_dt2/1 -> Mux/2
  Gain/1 -> Bus Creator/3  "u_bar"
  Bus Creator/1 -> inner_loop_indi/1  "inner_loop_indi"
  Control Allocation Vertical Acc Weighting/1(Delta_diag_W_v) -> INDI high level wls control allocation/7
  n_g_des/1 -> Control Allocation Vertical Acc Weighting/1(n_g_des)
  n_g/1 -> Control Allocation Vertical Acc Weighting/2(n_g)
  Is Manual Throttle Repmat/1(y) -> INDI high level wls control allocation/6
  Omega_Kb/1 -> control effectiveness/2(Omega_Kb)

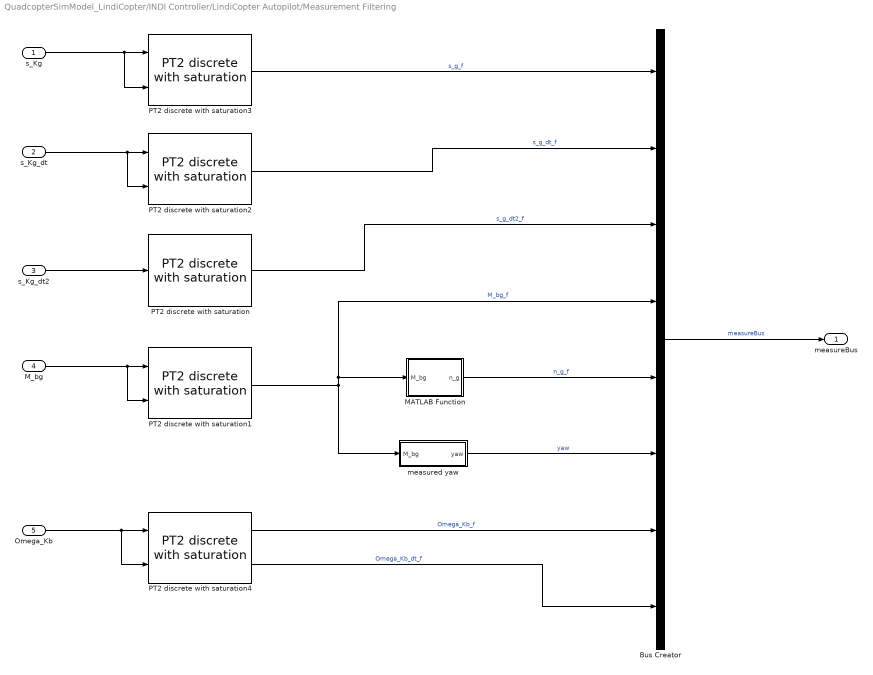
== system QuadcopterSimModel_LindiCopter/INDI Controller/LindiCopter Autopilot/Measurement Filtering ==
  s_Kg : Inport
  s_Kg_dt : Inport  Port=2
  s_Kg_dt2 : Inport  Port=3
  M_bg : Inport  Port=4
  Omega_Kb : Inport  Port=5
  Bus Creator : BusCreator  Inputs=8
  MATLAB Function : MATLAB Function  TreatAsAtomicUnit=on
  PT2 discrete with saturation : filters_lib/PT2 discrete with saturation  param_src=internal  omega=ap.sflt.omega  d=ap.sflt.D  x_dt2_max=inf  x_dt2_min=-inf  x_dt_max=inf  x_dt_min=-inf  x_max=inf  x_min=-inf  y_0_src=internal  x_init=0  y_dt_0_src=internal  x_dt_init=0  is_y_dt_checked=off  is_y_dt2_checked=off
      settings: SourceProductName=LADAC
  PT2 discrete with saturation1 : filters_lib/PT2 discrete with saturation  param_src=internal  omega=ap.sflt.omega  d=ap.sflt.D  x_dt2_max=inf  x_dt2_min=-inf  x_dt_max=inf  x_dt_min=-inf  x_max=inf  x_min=-inf  y_0_src=external  x_init=0  y_dt_0_src=internal  x_dt_init=0  is_y_dt_checked=off  is_y_dt2_checked=off
      settings: SourceProductName=LADAC
  PT2 discrete with saturation2 : filters_lib/PT2 discrete with saturation  param_src=internal  omega=ap.sflt.omega  d=ap.sflt.D  x_dt2_max=inf  x_dt2_min=-inf  x_dt_max=inf  x_dt_min=-inf  x_max=inf  x_min=-inf  y_0_src=external  x_init=0  y_dt_0_src=internal  x_dt_init=0  is_y_dt_checked=off  is_y_dt2_checked=off
      settings: SourceProductName=LADAC
  PT2 discrete with saturation3 : filters_lib/PT2 discrete with saturation  param_src=internal  omega=ap.sflt.omega  d=ap.sflt.D  x_dt2_max=inf  x_dt2_min=-inf  x_dt_max=inf  x_dt_min=-inf  x_max=inf  x_min=-inf  y_0_src=external  x_init=0  y_dt_0_src=internal  x_dt_init=0  is_y_dt_checked=off  is_y_dt2_checked=off
      settings: SourceProductName=LADAC
  PT2 discrete with saturation4 : filters_lib/PT2 discrete with saturation  param_src=internal  omega=ap.sflt.omega  d=ap.sflt.D  x_dt2_max=inf  x_dt2_min=-inf  x_dt_max=inf  x_dt_min=-inf  x_max=inf  x_min=-inf  y_0_src=external  x_init=0  y_dt_0_src=internal  x_dt_init=0  is_y_dt_checked=on  is_y_dt2_checked=off
      settings: SourceProductName=LADAC
  measured yaw : Subsystem
  measureBus : Outport
  wires:
  measured yaw/1(yaw) -> Bus Creator/6  "yaw"
  Bus Creator/1 -> measureBus/1  "measureBus"
  MATLAB Function/1(n_g) -> Bus Creator/5  "n_g_f"
  s_Kg/1 -> PT2 discrete with saturation3/1, PT2 discrete with saturation3/2
  PT2 discrete with saturation3/1 -> Bus Creator/1  "s_g_f"
  s_Kg_dt/1 -> PT2 discrete with saturation2/2, PT2 discrete with saturation2/1
  PT2 discrete with saturation2/1 -> Bus Creator/2  "s_g_dt_f"
  s_Kg_dt2/1 -> PT2 discrete with saturation/1
  PT2 discrete with saturation/1 -> Bus Creator/3  "s_g_dt2_f"
  PT2 discrete with saturation1/1 -> measured yaw/1(M_bg), Bus Creator/4, MATLAB Function/1(M_bg)  "M_bg_f"
  M_bg/1 -> PT2 discrete with saturation1/2, PT2 discrete with saturation1/1
  PT2 discrete with saturation4/1 -> Bus Creator/7  "Omega_Kb_f"
  Omega_Kb/1 -> PT2 discrete with saturation4/1, PT2 discrete with saturation4/2
  PT2 discrete with saturation4/2 -> Bus Creator/8  "Omega_Kb_dt_f"

== system QuadcopterSimModel_LindiCopter/INDI Controller/LindiCopter Autopilot/Pilot Reduced Attitude Commands ==
  stickCmdBus : Inport
  Enable : EnablePort
  Bus Creator : BusCreator  Inputs=4
  Bus Selector : BusSelector  OutputSignals=cmd_roll,cmd_pitch
  Gain : Gain  Gain=-1
  Gain1 : Gain  Gain=ap.atc.rm.leanmax
  MATLAB Function : MATLAB Function  TreatAsAtomicUnit=on
  MATLAB Function1 : MATLAB Function  TreatAsAtomicUnit=on
  red_atti_des : Outport
  wires:
  MATLAB Function/1(lean_angle) -> Gain1/1, Bus Creator/4  "cmd_lean_angle_0-1"
  Bus Creator/1 -> red_atti_des/1
  MATLAB Function1/1(n_g_des) -> Bus Creator/1  "n_g_des"
  Gain1/1 -> MATLAB Function1/1(lean_angle), Bus Creator/2  "lean_angle_des"
  MATLAB Function/2(lean_direction_angle) -> Bus Creator/3, MATLAB Function1/2(lean_dir_angle)  "lean_dir_angle_des"
  stickCmdBus/1 -> Bus Selector/1
  Bus Selector/2 -> Gain/1  "<cmd_pitch>"
  Bus Selector/1 -> MATLAB Function/1(stick_roll_cmd)  "<cmd_roll>"
  Gain/1 -> MATLAB Function/2(stick_pitch_cmd)

== system QuadcopterSimModel_LindiCopter/INDI Controller/LindiCopter Autopilot/State Logic Bus ==
  mode number : Inport
  is_traj_valid : Inport  Port=2
  LindiCopter State Logic : MATLAB Function  TreatAsAtomicUnit=on
  Unit Delay : UnitDelay  SampleTime=-1
  stateLogicBus : Outport
  wires:
  Unit Delay/1 -> LindiCopter State Logic/2(is_traj_valid)
  LindiCopter State Logic/1(state) -> stateLogicBus/1
  mode number/1 -> LindiCopter State Logic/1(mode_number)
  is_traj_valid/1 -> Unit Delay/1

== system QuadcopterSimModel_LindiCopter/INDI Controller/LindiCopter Autopilot/Stick Command Bus ==
  cmd_roll : Inport
  cmd_pitch : Inport  Port=2
  cmd_yaw : Inport  Port=3
  cmd_throttle : Inport  Port=4
  Bus Creator1 : BusCreator  Inputs=5
  throttle_-1_1 to throttle_0_1 : MATLAB Function  TreatAsAtomicUnit=on
  stickCmdBus : Outport
  wires:
  cmd_pitch/1 -> Bus Creator1/2
  cmd_throttle/1 -> Bus Creator1/4, throttle_-1_1 to throttle_0_1/1(throttle_m1_1)
  cmd_yaw/1 -> Bus Creator1/3
  Bus Creator1/1 -> stickCmdBus/1  "stickCmdBus"
  throttle_-1_1 to throttle_0_1/1(throttle_0_1) -> Bus Creator1/5  "cmd_throttle_0_1"
  cmd_roll/1 -> Bus Creator1/1

== system QuadcopterSimModel_LindiCopter/INDI Controller/LindiCopter Autopilot/Vertical Acc to Specific Thrust ==
  nu_z_g_dt2 : Inport
  M_bg_f : Inport  Port=2
  g : Inport  Port=3
  Enable : EnablePort
  Constant : Constant  Value=ap.psc.rm.accumax
  MATLAB Function : MATLAB Function  TreatAsAtomicUnit=on
  Selector : Selector  InputPortWidth=3  IndexOptions=Index vector (dialog)  Indices=3  OutputSizes=1
  T_spec_des : Outport
  wires:
  g/1 -> MATLAB Function/3(g)
  MATLAB Function/1(T_spec_des) -> T_spec_des/1
  M_bg_f/1 -> MATLAB Function/2(M_bg_f)
  nu_z_g_dt2/1 -> Selector/1
  Selector/1 -> MATLAB Function/1(nu_z_g_dt2)
  Constant/1 -> MATLAB Function/4(a_max)

== system QuadcopterSimModel_LindiCopter/INDI Controller/LindiCopter Autopilot/Copter Inner Loop INDI and Control Allocation/control effectiveness ==
  u : Inport
  Omega_Kb : Inport  Port=2
  Constant1 : Constant  Value=u_min
  MATLAB Function : MATLAB Function  TreatAsAtomicUnit=on
  Max : MinMax  Function=max  Inputs=2  OutDataTypeStr=Inherit: Inherit via back propagation
  G1 : Outport
  G2 : Outport  Port=2
  wires:
  u/1 -> Max/1
  Constant1/1 -> Max/2
  Max/1 -> MATLAB Function/1(u)
  MATLAB Function/1(G1) -> G1/1
  MATLAB Function/2(G2) -> G2/1
  Omega_Kb/1 -> MATLAB Function/2(Omega_Kb)

== system QuadcopterSimModel_LindiCopter/INDI Controller/LindiCopter Autopilot/Measurement Filtering/measured yaw ==
  M_bg : Inport
  DCM to quaternions : axes_transformation_lib/DCM to quaternions  SystemSampleTime=-1
      settings: SourceProductName=LADAC
  Quaternion Reduced : MATLAB Function  TreatAsAtomicUnit=on
  Terminator : Terminator
  yaw : Outport
  wires:
  M_bg/1 -> DCM to quaternions/1
  Quaternion Reduced/2(yaw) -> yaw/1  "yaw"
  Quaternion Reduced/1(q_red) -> Terminator/1
  DCM to quaternions/1 -> Quaternion Reduced/1(q_bg)

== matlab function QuadcopterSimModel_LindiCopter/INDI Controller/LindiCopter Autopilot/Measurement Filtering/MATLAB Function ==
  data: M_bg input; n_g output
function n_g = dcm2LeanVector( M_bg )
n_g = dcm2LeanVector( M_bg );
end

== matlab function QuadcopterSimModel_LindiCopter/INDI Controller/LindiCopter Autopilot/Copter Inner Loop INDI and Control Allocation/Control Allocation Vertical Acc Weighting ==
  data: n_g_des input; Delta_diag_W_v output; n_g input; ca parameter
function Delta_diag_W_v = caWlsCopterUpset(n_g_des,n_g,ca)
Delta_diag_W_v = caWlsCopterUpset(n_g_des,n_g,ca);
end

== matlab function QuadcopterSimModel_LindiCopter/INDI Controller/LindiCopter Autopilot/Pilot Reduced Attitude Commands/MATLAB Function ==
  data: stick_roll_cmd input; lean_angle output; stick_pitch_cmd input; lean_direction_angle output
function [lean_angle,lean_direction_angle] = fcn(stick_roll_cmd,stick_pitch_cmd)

lean_angle = sqrt( stick_roll_cmd^2 + stick_pitch_cmd^2 );
lean_direction_angle = atan2(stick_roll_cmd,-stick_pitch_cmd);

end

== matlab function QuadcopterSimModel_LindiCopter/INDI Controller/LindiCopter Autopilot/Pilot Reduced Attitude Commands/MATLAB Function1 ==
  data: lean_angle input; n_g_des output; lean_dir_angle input
function n_g_des = fcn(lean_angle,lean_dir_angle)

n_g_des = leanAngles2leanVector([lean_angle,lean_dir_angle]);

end

== matlab function QuadcopterSimModel_LindiCopter/INDI Controller/LindiCopter Autopilot/State Logic Bus/LindiCopter State Logic ==
  data: mode_number input; state output Bus: lindiStateLogicBus; is_traj_valid input
function state = lindiCopterStateLogic(mode_number, is_traj_valid)
state = lindiCopterStateLogic(mode_number,is_traj_valid);
end

== matlab function QuadcopterSimModel_LindiCopter/INDI Controller/LindiCopter Autopilot/Accelerations to Reduced Attitude and Thrust/MATLAB Function4 ==
  data: n_g input; phi output; delta output
function [phi,delta] = leanVector2LeanAngles(n_g)
[phi,delta] = leanVector2LeanAngles(n_g);
end

== matlab function QuadcopterSimModel_LindiCopter/INDI Controller/LindiCopter Autopilot/Vertical Acc to Specific Thrust/MATLAB Function ==
  data: nu_z_g_dt2 input; M_bg_f input; T_spec_des output; g input; a_max input
function T_spec_des = fcn(nu_z_g_dt2,M_bg_f,g,a_max)
den = M_bg_f(3,3);
T_spec_des = zeros(1,1,superiorfloat(nu_z_g_dt2(1)));
if den < g/a_max
    T_spec_des(:) = 0;
else
    T_spec_des(:) = divideFinite(-nu_z_g_dt2+g,den);
end
end

== matlab function QuadcopterSimModel_LindiCopter/INDI Controller/LindiCopter Autopilot/Stick Command Bus/throttle_-1_1 to throttle_0_1 ==
  data: throttle_m1_1 input; throttle_0_1 output
function throttle_0_1 = fcn(throttle_m1_1)
throttle_0_1 = 0.5*throttle_m1_1+0.5;

== matlab function QuadcopterSimModel_LindiCopter/INDI Controller/LindiCopter Autopilot/Copter Inner Loop INDI and Control Allocation/Is Manual Throttle Repmat ==
  data: u input; y output; ca parameter
function y = fcn(u,ca)
y = repmat(u,length(ca.u_d),1);
end

== matlab function QuadcopterSimModel_LindiCopter/INDI Controller/LindiCopter Autopilot/Copter Inner Loop INDI and Control Allocation/control effectiveness/MATLAB Function ==
  data: cep parameter; G10 parameter; G20 parameter; u input; G1 output; G2 output; Omega_Kb input
function [G1,G2] = indiCePropVar( cep, G10, G20, u,  Omega_Kb) %#codegen
[G1,G2] = indiCePropVar( cep, G10, G20, u, Omega_Kb );
end

== matlab function QuadcopterSimModel_LindiCopter/INDI Controller/LindiCopter Autopilot/Measurement Filtering/measured yaw/Quaternion Reduced ==
  data: q_bg input; q_red output; yaw output
function [q_red,yaw] = fcn(q_bg)
[q_red,yaw] = quatReduced(q_bg);
end
